simulink model "sampleModel327"  (R2021b)
settings: Solver=VariableStepAuto  StartTime=0.0  StopTime=10.0  RelTol=1e-3
undefined symbols (not defined in the file or in its folder): DiscIntNeverNeededParam, Newton, Raphson
libraries: simulink x18, simulink_need_slupdate x2
settings Model: Creator=user  LastModifiedBy=user

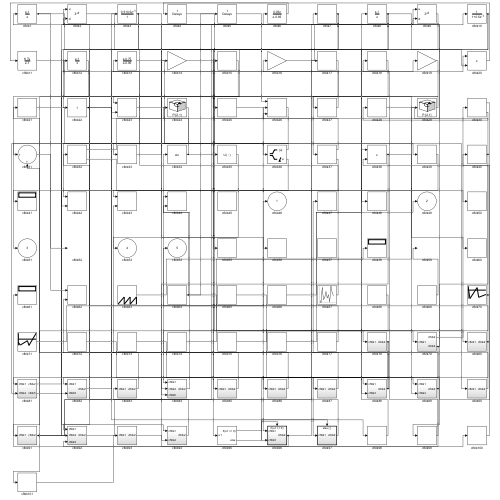
[thumbnail: Simulink's stored preview of the top-level diagram]
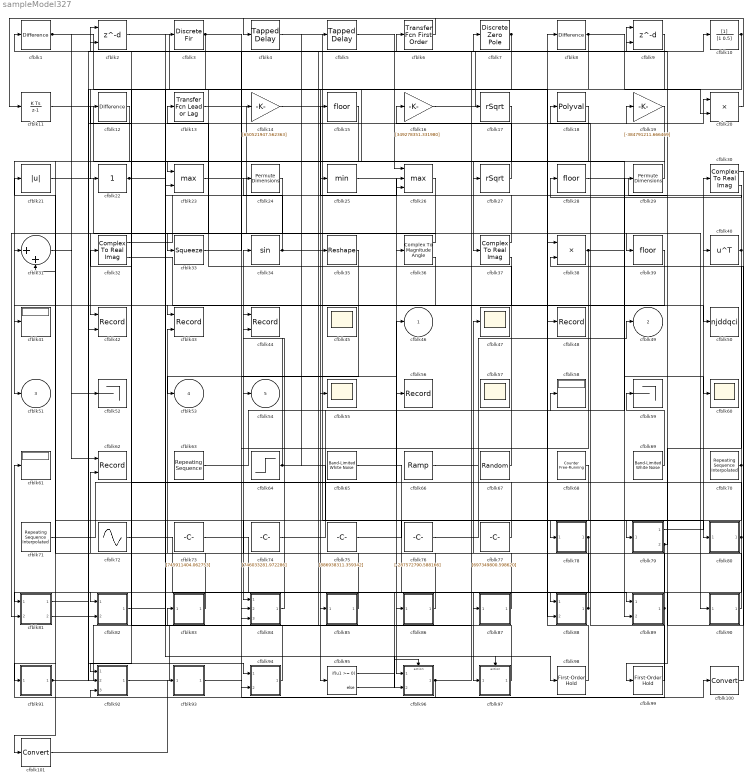
== system sampleModel327 ==
  cfblk1 : simulink/Discrete/Difference  ICPrevInput=0.0  OutMin=[]  OutMax=[]  OutDataTypeStr=Inherit: Inherit via back propagation  OutDataType=fixdt(1, 16)  OutScaling=2^-10  DoSatur=off
  cfblk10 : DiscreteFilter  SampleTime=1
  cfblk100 : DataTypeConversion
  cfblk101 : DataTypeConversion
  cfblk11 : DiscreteIntegrator  ICPrevOutput=DiscIntNeverNeededParam  ICPrevScaledInput=DiscIntNeverNeededParam
  cfblk12 : simulink/Discrete/Difference  ICPrevInput=0.0  OutMin=[]  OutMax=[]  OutDataTypeStr=Inherit: Inherit via back propagation  OutDataType=fixdt(1, 16)  OutScaling=2^-10  DoSatur=off
  cfblk13 : simulink/Discrete/Transfer Fcn Lead or Lag  PoleZ=0.95  ZeroZ=0.75  ICPrevOutput=0.0  ICPrevInput=0.0  DoSatur=off
      settings: SourceProductBaseCode=SL
  cfblk14 : Gain  Gain=[650521947.562363]
  cfblk15 : Rounding
  cfblk16 : Gain  Gain=[349278351.331980]
  cfblk17 : Sqrt  Operator=rSqrt  AlgorithmType=Newton-Raphson  SaturateOnIntegerOverflow=on
  cfblk18 : Polyval  Coefs=[ +2.081618890e-019, -1.441693666e-014, +4.719686976e-010, -8.536869453e-006, +1.621573104e-001, -8.087801117e+001 ]
  cfblk19 : Gain  Gain=[-384791211.666469]
  cfblk2 : Delay  DelayLengthSource=Input port  SampleTime=1
      settings: InputPortMap=u0,p1
  cfblk20 : Product  Inputs=**
  cfblk21 : Abs
  cfblk22 : simulink/Math Operations/Slider Gain  gain=1  low=0  high=2
  cfblk23 : MinMax  Function=max  Inputs=2
  cfblk24 : PermuteDimensions
  cfblk25 : MinMax
  cfblk26 : MinMax  Function=max  Inputs=3
  cfblk27 : Sqrt  Operator=rSqrt  AlgorithmType=Newton-Raphson  SaturateOnIntegerOverflow=on
  cfblk28 : Rounding
  cfblk29 : PermuteDimensions
  cfblk3 : DiscreteFir  SampleTime=1
  cfblk30 : ComplexToRealImag
  cfblk31 : Sum  Inputs=|++
  cfblk32 : ComplexToRealImag
  cfblk33 : Squeeze
  cfblk34 : Trigonometry
  cfblk35 : Reshape
  cfblk36 : ComplexToMagnitudeAngle
  cfblk37 : ComplexToRealImag
  cfblk38 : Product  Inputs=**
  cfblk39 : Rounding
  cfblk4 : simulink/Discrete/Tapped Delay  vinit=0.0  samptime=-1  NumDelays=1  DelayOrder=Oldest  includeCurrent=off
  cfblk40 : Math  Operator=transpose  SaturateOnIntegerOverflow=on
  cfblk41 : Display
  cfblk42 : Record  FileSettingsInternal="{\"entries\":[{\"content\":{\"excelSettings\":{\"content\":{},\"type\":\"Streamout.ExcelSettings\"}},\"type\":\"Streamout.FileSettingStorage\",\"uuid\":\"33c2ffa9-3b92-42b8-984e-0ea2b0a36ee0\"}],\"packageUris\":[\"http://schema.mathworks.com/mf0/streamout_blocks/R2020a\"],\"version\":\"1.0\"}"  Layout=[1 1]  SignalsInternal="{\"entries\":[{\"content\":{\"signals\":[{\"content\":{\"blockPath\":[\"sampleModel327/cfblk42\"],\"channel\":[],\"dimensions\":[1,1],\"domain\":\"sampleModel327/cfblk42\",\"lineColor\":\"#a2142f\",\"plots\":[1],\"port\":1,\"sid\":[\"\"],\"signalID\":13799,\"signalName\":\"cfblk24\"},\"type\":\"RecordBlkView.Signal\",\"uuid\":\"5bad4504-3fbc-4029-920c-c4ecb1b57935\"},{\"content\":{\"blockPath\":[\"sampleModel327/cfblk42\"],\"channel\":[],\"dimensions\":[1],\"domain\":\"sampleModel327/cfblk42\",\"lineColor\":\"#139fff\",\"plots\":[1],\"port\":2,\"sid\":[\"\"],\"signalID\":13803,\"signalName\":\"cfblk39\"},\"type\":\"RecordBlkView.Signal\",\"uuid\":\"ec51d72b-9738-4f64-9b7e-5afc926f3a9a\"}]},\"type\":\"RecordBlkView.InputSignals\",\"uuid\":\"7e7397b2-d1cb-4ab5-85cf-9b07b568169d\"}],\"packageUris\":[\"http://schema.mathworks.com/mf0/streamout_blocks/R2020a\"],\"version\":\"1.0\"}"  VisualizationBindings="{\"xyplotplugin\":{\"info\":[{\"series\":[{\"bindingParametersList\":[{\"parameter\":\"X-Axis\",\"signalID\":13799,\"signalName\":\"cfblk24\"},{\"parameter\":\"Y-Axis\",\"signalID\":13803,\"signalName\":\"cfblk39\"}],\"seriesID\":61504}],\"subplotID\":1}]}}"  CompatibilityTag=XY
  cfblk43 : Record  FileSettingsInternal="{\"entries\":[{\"content\":{\"excelSettings\":{\"content\":{},\"type\":\"Streamout.ExcelSettings\"}},\"type\":\"Streamout.FileSettingStorage\",\"uuid\":\"75856b50-8802-40e8-b79a-6243b943a5fc\"}],\"packageUris\":[\"http://schema.mathworks.com/mf0/streamout_blocks/R2020a\"],\"version\":\"1.0\"}"  Layout=[1 1]  SignalsInternal="{\"entries\":[{\"content\":{\"signals\":[{\"content\":{\"blockPath\":[\"sampleModel327/cfblk43\"],\"channel\":[],\"dimensions\":[1],\"domain\":\"sampleModel327/cfblk43\",\"lineColor\":\"#a2142f\",\"plots\":[1],\"port\":1,\"sid\":[\"\"],\"signalID\":13807,\"signalName\":\"cfblk36:2\"},\"type\":\"RecordBlkView.Signal\",\"uuid\":\"e75b9d34-f0aa-46d9-8ef1-c5efd0b51d10\"},{\"content\":{\"blockPath\":[\"sampleModel327/cfblk43\"],\"channel\":[],\"dimensions\":[1],\"domain\":\"sampleModel327/cfblk43\",\"lineColor\":\"#139fff\",\"plots\":[1],\"port\":2,\"sid\":[\"\"],\"signalID\":13811,\"signalName\":\"cfblk83\"},\"type\":\"RecordBlkView.Signal\",\"uuid\":\"494e2e49-f910-4ea1-b2cc-9eb513637dbe\"}]},\"type\":\"RecordBlkView.InputSignals\",\"uuid\":\"3fc81e13-d54e-422d-9697-93ffdd8bb91f\"}],\"packageUris\":[\"http://schema.mathworks.com/mf0/streamout_blocks/R2020a\"],\"version\":\"1.0\"}"  VisualizationBindings="{\"xyplotplugin\":{\"info\":[{\"series\":[{\"bindingParametersList\":[{\"parameter\":\"X-Axis\",\"signalID\":13807,\"signalName\":\"cfblk36:2\"},{\"parameter\":\"Y-Axis\",\"signalID\":13811,\"signalName\":\"cfblk83\"}],\"seriesID\":32840}],\"subplotID\":1}]}}"  CompatibilityTag=XY
  cfblk44 : Record  FileSettingsInternal="{\"entries\":[{\"content\":{\"excelSettings\":{\"content\":{},\"type\":\"Streamout.ExcelSettings\"}},\"type\":\"Streamout.FileSettingStorage\",\"uuid\":\"ef7e7a48-7fda-4d4e-948c-ba98d64ff4e2\"}],\"packageUris\":[\"http://schema.mathworks.com/mf0/streamout_blocks/R2020a\"],\"version\":\"1.0\"}"  Layout=[1 1]  SignalsInternal="{\"entries\":[{\"content\":{\"signals\":[{\"content\":{\"blockPath\":[\"sampleModel327/cfblk44\"],\"channel\":[],\"dimensions\":[1],\"domain\":\"sampleModel327/cfblk44\",\"lineColor\":\"#a2142f\",\"plots\":[1],\"port\":1,\"sid\":[\"\"],\"signalID\":13815,\"signalName\":\"cfblk64\"},\"type\":\"RecordBlkView.Signal\",\"uuid\":\"76e43ab0-c2b9-4fb9-8d83-66e50747795d\"},{\"content\":{\"blockPath\":[\"sampleModel327/cfblk44\"],\"channel\":[],\"dimensions\":[1],\"domain\":\"sampleModel327/cfblk44\",\"lineColor\":\"#139fff\",\"plots\":[1],\"port\":2,\"sid\":[\"\"],\"signalID\":13819,\"signalName\":\"cfblk84\"},\"type\":\"RecordBlkView.Signal\",\"uuid\":\"477e6fc5-5fd6-414f-aede-7285462d46db\"}]},\"type\":\"RecordBlkView.InputSignals\",\"uuid\":\"526753ab-ad5c-4902-a3af-d1b50829fbdf\"}],\"packageUris\":[\"http://schema.mathworks.com/mf0/streamout_blocks/R2020a\"],\"version\":\"1.0\"}"  VisualizationBindings="{\"xyplotplugin\":{\"info\":[{\"series\":[{\"bindingParametersList\":[{\"parameter\":\"X-Axis\",\"signalID\":13815,\"signalName\":\"cfblk64\"},{\"parameter\":\"Y-Axis\",\"signalID\":13819,\"signalName\":\"cfblk84\"}],\"seriesID\":24490}],\"subplotID\":1}]}}"  CompatibilityTag=XY
  cfblk{45,47,55,57,60} (5 alike) : Scope
      cfblk45 settings: Floating=on
      cfblk57 settings: Floating=on
  cfblk48 : Record  FileSettingsInternal="{\"entries\":[{\"content\":{\"excelSettings\":{\"content\":{},\"type\":\"Streamout.ExcelSettings\"}},\"type\":\"Streamout.FileSettingStorage\",\"uuid\":\"ade0aac1-33e1-4039-bb3e-e289e615a570\"}],\"packageUris\":[\"http://schema.mathworks.com/mf0/streamout_blocks/R2020a\"],\"version\":\"1.0\"}"  SignalsInternal="{\"entries\":[{\"content\":{\"signals\":[{\"content\":{\"blockPath\":[\"sampleModel327/cfblk48\"],\"channel\":[],\"dimensions\":[1],\"domain\":\"sampleModel327/cfblk48\",\"lineColor\":\"#b746ff\",\"plots\":[1],\"port\":1,\"sid\":[\"\"],\"signalID\":13823,\"signalName\":\"cfblk1\"},\"type\":\"RecordBlkView.Signal\",\"uuid\":\"edf4636b-a3ed-4be5-b103-aafec9c72770\"}]},\"type\":\"RecordBlkView.InputSignals\",\"uuid\":\"02883b60-b2fa-4de9-bc2e-2ff48d54d8c4\"}],\"packageUris\":[\"http://schema.mathworks.com/mf0/streamout_blocks/R2020a\"],\"version\":\"1.0\"}"  VisualizationBindings="{\"sparklinesplugin\":{\"info\":[{\"bindingParametersList\":[],\"subplotID\":1}]}}"
  cfblk5 : simulink/Discrete/Tapped Delay  vinit=0.0  samptime=-1  NumDelays=1  DelayOrder=Oldest  includeCurrent=off
  cfblk50 : ToWorkspace  VariableName=njddqci  SaveFormat=Timeseries  SampleTime=-1
  cfblk52 : Terminator
  cfblk56 : Record  FileSettingsInternal="{\"entries\":[{\"content\":{\"excelSettings\":{\"content\":{},\"type\":\"Streamout.ExcelSettings\"}},\"type\":\"Streamout.FileSettingStorage\",\"uuid\":\"41e1043c-8eaf-4d4e-a378-7d19dd63403e\"}],\"packageUris\":[\"http://schema.mathworks.com/mf0/streamout_blocks/R2020a\"],\"version\":\"1.0\"}"  SignalsInternal="{\"entries\":[{\"content\":{\"signals\":[{\"content\":{\"blockPath\":[\"sampleModel327/cfblk56\"],\"channel\":[],\"dimensions\":[1],\"domain\":\"sampleModel327/cfblk56\",\"lineColor\":\"#64d413\",\"plots\":[1],\"port\":1,\"sid\":[\"\"],\"signalID\":13827,\"signalName\":\"cfblk3\"},\"type\":\"RecordBlkView.Signal\",\"uuid\":\"78df5ed0-a601-4abd-8e36-a9342c828ac9\"}]},\"type\":\"RecordBlkView.InputSignals\",\"uuid\":\"fc51c003-aacf-4840-975e-d844f08af6c5\"}],\"packageUris\":[\"http://schema.mathworks.com/mf0/streamout_blocks/R2020a\"],\"version\":\"1.0\"}"  VisualizationBindings="{\"sparklinesplugin\":{\"info\":[{\"bindingParametersList\":[],\"subplotID\":1}]}}"
  cfblk58 : Display
  cfblk59 : Terminator
  cfblk6 : simulink/Discrete/Transfer Fcn First Order  PoleZ=0.95  ICPrevOutput=0.0  DoSatur=off
  cfblk61 : Display
  cfblk62 : Record  FileSettingsInternal="{\"entries\":[{\"content\":{\"excelSettings\":{\"content\":{},\"type\":\"Streamout.ExcelSettings\"}},\"type\":\"Streamout.FileSettingStorage\",\"uuid\":\"cf0e630a-b6ea-4c08-9722-0a847d5db507\"}],\"packageUris\":[\"http://schema.mathworks.com/mf0/streamout_blocks/R2020a\"],\"version\":\"1.0\"}"  Layout=[1 1]  SignalsInternal="{\"entries\":[{\"content\":{\"signals\":[{\"content\":{\"blockPath\":[\"sampleModel327/cfblk62\"],\"channel\":[],\"dimensions\":[1],\"domain\":\"sampleModel327/cfblk62\",\"lineColor\":\"#a2142f\",\"plots\":[1],\"port\":1,\"sid\":[\"\"],\"signalID\":13831,\"signalName\":\"cfblk31\"},\"type\":\"RecordBlkView.Signal\",\"uuid\":\"77f17b6b-0617-4a7a-923e-7f2136a48b06\"},{\"content\":{\"blockPath\":[\"sampleModel327/cfblk62\"],\"channel\":[],\"dimensions\":[1,1],\"domain\":\"sampleModel327/cfblk62\",\"lineColor\":\"#139fff\",\"plots\":[1],\"port\":2,\"sid\":[\"\"],\"signalID\":13835,\"signalName\":\"cfblk89\"},\"type\":\"RecordBlkView.Signal\",\"uuid\":\"eb02ab39-edf6-4666-a4af-b852e5bb6c4a\"}]},\"type\":\"RecordBlkView.InputSignals\",\"uuid\":\"c8cb87dc-5242-41ef-a874-03461642eaf9\"}],\"packageUris\":[\"http://schema.mathworks.com/mf0/streamout_blocks/R2020a\"],\"version\":\"1.0\"}"  VisualizationBindings="{\"xyplotplugin\":{\"info\":[{\"series\":[{\"bindingParametersList\":[{\"parameter\":\"X-Axis\",\"signalID\":13831,\"signalName\":\"cfblk31\"},{\"parameter\":\"Y-Axis\",\"signalID\":13835,\"signalName\":\"cfblk89\"}],\"seriesID\":20513}],\"subplotID\":1}]}}"  CompatibilityTag=XY
  cfblk63 : simulink/Sources/Repeating Sequence  rep_seq_t=[0 2]  rep_seq_y=[-295941772.283412, -181536480.920542]
  cfblk64 : Step  Time=[26.000000]  Before=[787564212.823436]  After=[272902529.416691]  SampleTime=0
  cfblk65 : simulink/Sources/Band-Limited White Noise  Cov=[2107124818.535533]  Ts=0.1  seed=[9975265161.000000]
  cfblk66 : simulink/Sources/Ramp  slope=[1189.066786]  start=[14.665538]  InitialOutput=[-279965.942118]
  cfblk67 : UniformRandomNumber  Minimum=[-4913656888.347259]  Maximum=[2983539929.867875]  Seed=[56800548.000000]  SampleTime=0.1
  cfblk68 : simulink/Sources/Counter Free-Running  NumBits=[16.000000]  tsamp=-1
  cfblk69 : simulink/Sources/Band-Limited White Noise  Cov=[134068197.174960]  Ts=0.1  seed=[8416163319.000000]
  cfblk7 : DiscreteZeroPole  Poles=[0 0.5]  Gain=1
  cfblk70 : simulink/Sources/Repeating Sequence Interpolated  OutValues=[390093350.816152, -880915595.683774, 254144513.360107, -776097889.307030, -452323757.197211]  TimeValues=[0 0.1 0.5 0.6 1].'  LookUpMeth=Use Input Below  tsamp=0.01  OutMin=[]  OutMax=[]  OutDataTypeStr=double  OutputDataTypeScalingMode=double  OutDataType=fixdt(0,8)  OutScaling=2^-10
  cfblk71 : simulink/Sources/Repeating Sequence Interpolated  OutValues=[-433490176.727405, -810040466.549954, -214148032.514127, -828178424.658375, 820853163.486793]  TimeValues=[0 0.1 0.5 0.6 1].'  LookUpMeth=Use Input Nearest  tsamp=0.01  OutMin=[]  OutMax=[]  OutDataTypeStr=double  OutputDataTypeScalingMode=double  OutDataType=fixdt(0,8)  OutScaling=2^-10
  cfblk72 : Sin  Amplitude=[-354076390.408575]  Bias=[138076503.488791]  SampleTime=0
  cfblk73 : Constant  Value=[745911404.062753]  SampleTime=1
  cfblk74 : Constant  Value=[746033281.972286]  SampleTime=1
  cfblk75 : Constant  Value=[886938311.359342]  SampleTime=1
  cfblk76 : Constant  Value=[-287572790.588166]  SampleTime=1
  cfblk77 : Constant  Value=[697349800.598620]  SampleTime=1
  cfblk78 : Subsystem
  cfblk79 : Subsystem
  cfblk8 : simulink/Discrete/Difference  ICPrevInput=0.0  OutMin=[]  OutMax=[]  OutDataTypeStr=Inherit: Inherit via back propagation  OutDataType=fixdt(1, 16)  OutScaling=2^-10  DoSatur=off
  cfblk80 : Subsystem
  cfblk81 : Subsystem
  cfblk82 : Subsystem
  cfblk83 : Subsystem
  cfblk84 : Subsystem
  cfblk85 : Subsystem
  cfblk86 : Subsystem
  cfblk87 : Subsystem
  cfblk88 : Subsystem
  cfblk89 : Subsystem
  cfblk9 : Delay  DelayLengthSource=Input port  SampleTime=1
      settings: InputPortMap=u0,p1
  cfblk90 : Subsystem
  cfblk91 : Subsystem
  cfblk92 : Subsystem
  cfblk93 : Subsystem
  cfblk94 : Subsystem
  cfblk95 : If  IfExpression=u1 >= 0  SampleTime=1
  cfblk96 : Subsystem  TreatAsAtomicUnit=on
  cfblk97 : Subsystem  TreatAsAtomicUnit=on
  cfblk98 : simulink_need_slupdate/First-Order Hold  DisableCoverage=on  Ts=1
      settings: SourceProductBaseCode=SL
  cfblk99 : simulink_need_slupdate/First-Order Hold  DisableCoverage=on  Ts=1
      settings: SourceProductBaseCode=SL
  cfblk46 : Outport
  cfblk49 : Outport  Port=2
  cfblk51 : Outport  Port=3
  cfblk53 : Outport  Port=4
  cfblk54 : Outport  Port=5
  wires:
  cfblk24/1 -> cfblk42/1
  cfblk29/1 -> cfblk23/1
  cfblk14/1 -> cfblk78/1(cfblk1)
  cfblk90/1(cfblk2) -> cfblk32/1
  cfblk28/1 -> cfblk1/1
  cfblk19/1 -> cfblk37/1
  cfblk25/1 -> cfblk96/1(cfblk1)
  cfblk89/1(cfblk2) -> cfblk61/1, cfblk62/2
  cfblk22/1 -> cfblk26/3, cfblk98/1
  cfblk77/1 -> cfblk34/1
  cfblk30/1 -> cfblk97/1(cfblk1)
  cfblk94/1(cfblk2) -> cfblk83/1(cfblk1)
  cfblk30/2 -> cfblk28/1
  cfblk16/1 -> cfblk9/1
  cfblk21/1 -> cfblk39/1
  cfblk65/1 -> cfblk87/1(cfblk1)
  cfblk66/1 -> cfblk8/1
  cfblk18/1 -> cfblk51/1
  cfblk73/1 -> cfblk88/1(cfblk1)
  cfblk67/1 -> cfblk13/1
  cfblk13/1 -> cfblk95/1
  cfblk17/1 -> cfblk27/1
  cfblk79/1(cfblk2) -> cfblk30/1
  cfblk88/1(cfblk2) -> cfblk82/1(cfblk1), cfblk31/2
  cfblk4/1 -> cfblk36/1
  cfblk7/1 -> cfblk22/1, cfblk94/2(cfblk4)
  cfblk96/1(cfblk2) -> cfblk9/2, cfblk92/3(cfblk5)
  cfblk72/1 -> cfblk89/1(cfblk1)
  cfblk86/1(cfblk2) -> cfblk54/1
  cfblk64/1 -> cfblk44/1, cfblk5/1, cfblk79/1(cfblk1)
  cfblk69/1 -> cfblk59/1
  cfblk78/1(cfblk2) -> cfblk96/2(cfblk3), cfblk84/2(cfblk4)
  cfblk71/1 -> cfblk46/1
  cfblk11/1 -> cfblk89/2(cfblk4)
  cfblk31/1 -> cfblk62/1
  cfblk12/1 -> cfblk82/2(cfblk5)
  cfblk63/1 -> cfblk58/1
  cfblk97/1(cfblk2) -> cfblk12/1
  cfblk82/1(cfblk2) -> cfblk19/1
  cfblk79/2(cfblk4) -> cfblk86/1(cfblk1), cfblk2/2
  cfblk2/1 -> cfblk85/1(cfblk1)
  cfblk84/1(cfblk2) -> cfblk44/2
  cfblk9/1 -> cfblk55/1
  cfblk39/1 -> cfblk42/2
  cfblk36/1 -> cfblk31/1
  cfblk10/1 -> cfblk88/2(cfblk3), cfblk92/2(cfblk4)
  cfblk70/1 -> cfblk18/1, cfblk84/1(cfblk1)
  cfblk85/1(cfblk2) -> cfblk21/1
  cfblk36/2 -> cfblk43/1
  cfblk83/1(cfblk2) -> cfblk43/2
  cfblk37/1 -> cfblk15/1
  cfblk33/1 -> cfblk6/1
  cfblk1/1 -> cfblk48/1, cfblk52/1
  cfblk92/1(cfblk2) -> cfblk35/1
  cfblk8/1 -> cfblk33/1, cfblk25/1, cfblk20/2
  cfblk15/1 -> cfblk81/1(cfblk1)
  cfblk87/1(cfblk2) -> cfblk47/1
  cfblk75/1 -> cfblk80/1(cfblk1)
  cfblk91/1(cfblk2) -> cfblk17/1, cfblk3/1, cfblk10/1
  cfblk26/1 -> cfblk81/2(cfblk4)
  cfblk20/1 -> cfblk11/1
  cfblk3/1 -> cfblk23/2, cfblk56/1, cfblk92/1(cfblk1)
  cfblk37/2 -> cfblk41/1
  cfblk23/1 -> cfblk90/1(cfblk1)
  cfblk34/1 -> cfblk24/1, cfblk7/1
  cfblk32/1 -> cfblk14/1
  cfblk40/1 -> cfblk26/2, cfblk99/1
  cfblk32/2 -> cfblk50/1
  cfblk38/1 -> cfblk60/1, cfblk84/3(cfblk5)
  cfblk74/1 -> cfblk29/1
  cfblk35/1 -> cfblk53/1
  cfblk5/1 -> cfblk26/1
  cfblk6/1 -> cfblk4/1
  cfblk81/1(cfblk2) -> cfblk20/1
  cfblk27/1 -> cfblk16/1
  cfblk81/2(cfblk5) -> cfblk94/1(cfblk1)
  cfblk80/1(cfblk2) -> cfblk91/1(cfblk1), cfblk2/1
  cfblk76/1 -> cfblk49/1
  cfblk95/1 -> cfblk96/Action
  cfblk95/2 -> cfblk97/Action
  cfblk98/1 -> cfblk38/1
  cfblk99/1 -> cfblk38/2
  cfblk93/1(cfblk2) -> cfblk100/1
  cfblk100/1 -> cfblk40/1
  cfblk68/1 -> cfblk101/1
  cfblk101/1 -> cfblk93/1(cfblk1)

== system sampleModel327/cfblk78 ==
  cfblk1 : Inport
  cfblk3 : Polyval  Coefs=[ +2.081618890e-019, -1.441693666e-014, +4.719686976e-010, -8.536869453e-006, +1.621573104e-001, -8.087801117e+001 ]
  cfblk2 : Outport
  wires:
  cfblk3/1 -> cfblk2/1
  cfblk1/1 -> cfblk3/1

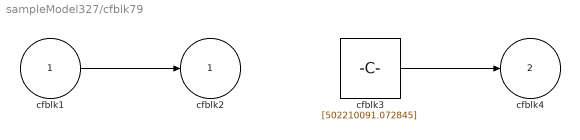
== system sampleModel327/cfblk79 ==
  cfblk1 : Inport
  cfblk3 : Constant  Value=[502210091.072845]  SampleTime=1
  cfblk2 : Outport
  cfblk4 : Outport  Port=2
  wires:
  cfblk3/1 -> cfblk4/1
  cfblk1/1 -> cfblk2/1

== system sampleModel327/cfblk80 ==
  cfblk1 : Inport
  cfblk3 : Delay  SampleTime=1
  cfblk2 : Outport
  wires:
  cfblk1/1 -> cfblk3/1
  cfblk3/1 -> cfblk2/1

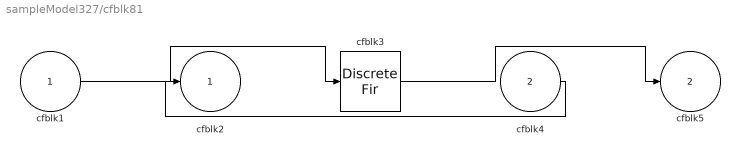
== system sampleModel327/cfblk81 ==
  cfblk1 : Inport
  cfblk4 : Inport  Port=2
  cfblk3 : DiscreteFir  SampleTime=1
  cfblk2 : Outport
  cfblk5 : Outport  Port=2
  wires:
  cfblk1/1 -> cfblk3/1
  cfblk4/1 -> cfblk2/1
  cfblk3/1 -> cfblk5/1

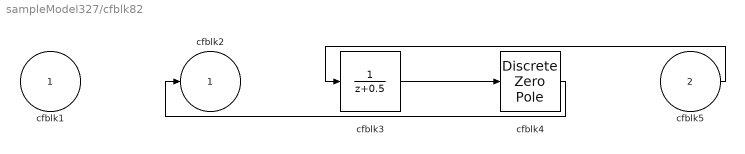
== system sampleModel327/cfblk82 ==
  cfblk1 : Inport
  cfblk5 : Inport  Port=2
  cfblk3 : DiscreteTransferFcn  SampleTime=1
  cfblk4 : DiscreteZeroPole  Poles=[0 0.5]  Gain=1
  cfblk2 : Outport
  wires:
  cfblk3/1 -> cfblk4/1
  cfblk5/1 -> cfblk3/1
  cfblk4/1 -> cfblk2/1

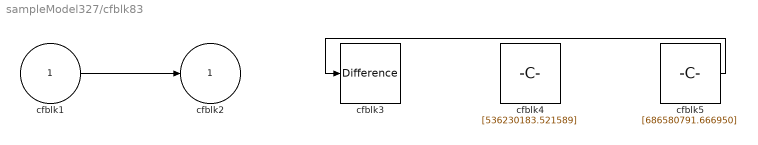
== system sampleModel327/cfblk83 ==
  cfblk1 : Inport
  cfblk3 : simulink/Discrete/Difference  ICPrevInput=0.0  OutMin=[]  OutMax=[]  OutDataTypeStr=Inherit: Inherit via back propagation  OutDataType=fixdt(1, 16)  OutScaling=2^-10  DoSatur=off
  cfblk4 : Constant  Value=[536230183.521589]  SampleTime=1
  cfblk5 : Constant  Value=[686580791.666950]  SampleTime=1
  cfblk2 : Outport
  wires:
  cfblk1/1 -> cfblk2/1
  cfblk5/1 -> cfblk3/1

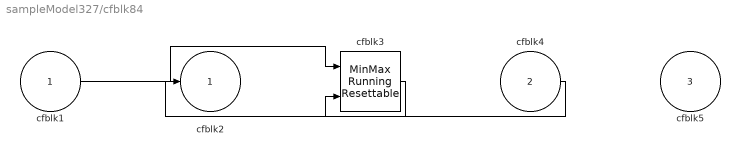
== system sampleModel327/cfblk84 ==
  cfblk1 : Inport
  cfblk4 : Inport  Port=2
  cfblk5 : Inport  Port=3
  cfblk3 : simulink/Math Operations/MinMax Running Resettable  Function=min  vinit=0.0
  cfblk2 : Outport
  wires:
  cfblk1/1 -> cfblk3/1
  cfblk3/1 -> cfblk2/1
  cfblk4/1 -> cfblk3/2

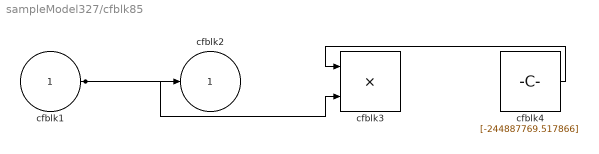
== system sampleModel327/cfblk85 ==
  cfblk1 : Inport
  cfblk3 : Product
  cfblk4 : Constant  Value=[-244887769.517866]  SampleTime=1
  cfblk2 : Outport
  wires:
  cfblk1/1 -> cfblk2/1, cfblk3/2
  cfblk4/1 -> cfblk3/1

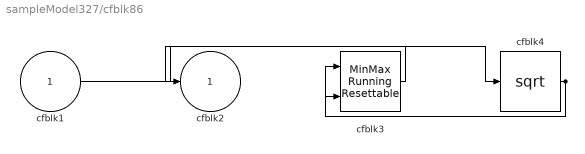
== system sampleModel327/cfblk86 ==
  cfblk1 : Inport
  cfblk3 : simulink/Math Operations/MinMax Running Resettable  Function=min  vinit=0.0
  cfblk4 : Sqrt  SaturateOnIntegerOverflow=on
  cfblk2 : Outport
  wires:
  cfblk1/1 -> cfblk4/1
  cfblk4/1 -> cfblk3/1, cfblk3/2
  cfblk3/1 -> cfblk2/1

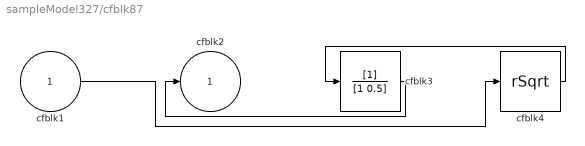
== system sampleModel327/cfblk87 ==
  cfblk1 : Inport
  cfblk3 : DiscreteFilter  SampleTime=1
  cfblk4 : Sqrt  Operator=rSqrt  AlgorithmType=Newton-Raphson  SaturateOnIntegerOverflow=on
  cfblk2 : Outport
  wires:
  cfblk4/1 -> cfblk3/1
  cfblk3/1 -> cfblk2/1
  cfblk1/1 -> cfblk4/1

== system sampleModel327/cfblk88 ==
  cfblk1 : Inport
  cfblk3 : Inport  Port=2
  cfblk2 : Outport
  wires:
  cfblk1/1 -> cfblk2/1

== system sampleModel327/cfblk89 ==
  cfblk1 : Inport
  cfblk4 : Inport  Port=2
  cfblk3 : Delay  SampleTime=1
  cfblk2 : Outport
  wires:
  cfblk4/1 -> cfblk2/1
  cfblk1/1 -> cfblk3/1

== system sampleModel327/cfblk90 ==
  cfblk1 : Inport
  cfblk3 : Bias  Bias=[-849613791.759812]
  cfblk2 : Outport
  wires:
  cfblk1/1 -> cfblk3/1
  cfblk3/1 -> cfblk2/1

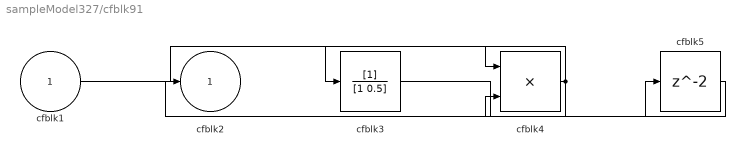
== system sampleModel327/cfblk91 ==
  cfblk1 : Inport
  cfblk3 : DiscreteFilter  SampleTime=1
  cfblk4 : Product
  cfblk5 : Delay  SampleTime=1
  cfblk2 : Outport
  wires:
  cfblk1/1 -> cfblk4/1
  cfblk4/1 -> cfblk2/1, cfblk3/1
  cfblk3/1 -> cfblk5/1
  cfblk5/1 -> cfblk4/2

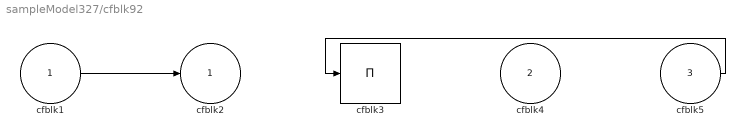
== system sampleModel327/cfblk92 ==
  cfblk1 : Inport
  cfblk4 : Inport  Port=2
  cfblk5 : Inport  Port=3
  cfblk3 : Product  Inputs=*
  cfblk2 : Outport
  wires:
  cfblk1/1 -> cfblk2/1
  cfblk5/1 -> cfblk3/1

== system sampleModel327/cfblk93 ==
  cfblk1 : Inport
  cfblk3 : DiscreteTransferFcn  SampleTime=1
  cfblk2 : Outport
  wires:
  cfblk1/1 -> cfblk2/1, cfblk3/1

== system sampleModel327/cfblk94 ==
  cfblk1 : Inport
  cfblk4 : Inport  Port=2
  cfblk3 : UnitDelay  HasFrameUpgradeWarning=on
  cfblk2 : Outport
  wires:
  cfblk4/1 -> cfblk3/1
  cfblk3/1 -> cfblk2/1

== system sampleModel327/cfblk96 ==
  cfblk1 : Inport
  cfblk3 : Inport  Port=2
  Action Port : ActionPort  ActionPortLabel=if(u1 >= 0)
  cfblk2 : Outport
  wires:
  cfblk1/1 -> cfblk2/1

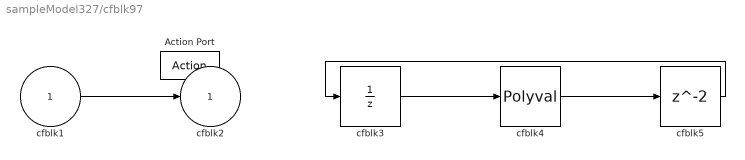
== system sampleModel327/cfblk97 ==
  cfblk1 : Inport
  Action Port : ActionPort  ActionPortLabel=else
  cfblk3 : UnitDelay  SampleTime=-1  HasFrameUpgradeWarning=on
  cfblk4 : Polyval  Coefs=[ +2.081618890e-019, -1.441693666e-014, +4.719686976e-010, -8.536869453e-006, +1.621573104e-001, -8.087801117e+001 ]
  cfblk5 : Delay
  cfblk2 : Outport
  wires:
  cfblk3/1 -> cfblk4/1
  cfblk1/1 -> cfblk2/1
  cfblk4/1 -> cfblk5/1
  cfblk5/1 -> cfblk3/1
